simulink model "BuckyWagon_01"  (Simulink 7.5)
settings: Solver=FixedStepDiscrete  StartTime=0.0  StopTime=10.0  RelTol=1e-3
PreLoadFcn:
  | try, eval([bdroot '_setup']); catch, eval('model_setup', ''); end
InitFcn:
  | try, eval([bdroot '_setup']); catch, eval('model_setup', ''); end
undefined symbols (not defined in the file): ECU565, High, Low, miniviewSetup, motohawk_build_version, motohawk_get_faults, motohawk_setup_toolchains, motohawk_trunc_name, motohawk_vardec_config_group, motohawk_vardec_path, tc, True
libraries: MotoHawk_lib x381, simulink x26, miniview_lib x10, motohawk_control_primitives_lib x8, motohawk_engine_lib x6, motohawk_annotations_lib x2
(part 3 of 6)

== system BuckyWagon_01/Strategy/Actuators/A123 Battery Controller ==
  Contactor Command : Inport  OutDataType=sfix(16)  OutScaling=2^0
  Compare To Constant : simulink/Logic and Bit Operations/Compare To Constant  SystemSampleTime=-1  relop=>=  const=5  LogicOutDataTypeMode=uint8
  Emergency Power Off Comand : Constant  Value=0  OutDataTypeMode=uint8  OutDataType=fixdt(1, 16)  OutScaling=2^0  OutDataTypeStr=uint8
  Main Enable : Constant  OutDataTypeMode=uint8  OutDataType=fixdt(1, 16)  OutScaling=2^0  OutDataTypeStr=uint8
  Send CAN Messages3 : MotoHawk_lib/CAN Blocks/Send CAN Messages  bus=-2  nam='CAN_2'  msgl=BMS_A123_400  pace=5  labelwires=off
  Time Since Enabled (With Input)1 : motohawk_control_primitives_lib/Time Since Enabled (With Input)1  SystemSampleTime=-1  nam='A123_GroundFaultDetector_Enable_Timer'  samp_time=-1  init=0  upperlim=3600*24
  motohawk_override_abs5 : MotoHawk_lib/Calibration & Probing Blocks/motohawk_override_abs  SystemSampleTime=-1  parent_name='hsc_bcm_enable'  parent_val=0  show_more=on  name_source=Use Parameter  parent_read_level=1  parent_override_level=1  view_as=Number  enum_struct={'Disabled', 'Enabled'}  use_help_units=off  parent_help=''  parent_units=''  use_min_max=off  parent_min=-inf  parent_max=inf  use_precision=off  parent_precision=''  parent_gain=1  parent_offset=0  parent_exp=1  use_mototune_group=on  parent_group='Actuators | BCM'
  motohawk_override_abs6 : MotoHawk_lib/Calibration & Probing Blocks/motohawk_override_abs  SystemSampleTime=-1  parent_name='hsc_bcm_epo'  parent_val=0  show_more=on  name_source=Use Parameter  parent_read_level=1  parent_override_level=1  view_as=Number  enum_struct={'Disabled', 'Enabled'}  use_help_units=off  parent_help=''  parent_units=''  use_min_max=off  parent_min=-inf  parent_max=inf  use_precision=off  parent_precision=''  parent_gain=1  parent_offset=0  parent_exp=1  use_mototune_group=on  parent_group='Actuators | BCM'
  motohawk_override_abs7 : MotoHawk_lib/Calibration & Probing Blocks/motohawk_override_abs  SystemSampleTime=-1  parent_name='hsc_bcm_leakage_enable'  parent_val=0  show_more=on  name_source=Use Parameter  parent_read_level=1  parent_override_level=1  view_as=Number  enum_struct={'Disabled', 'Enabled'}  use_help_units=off  parent_help=''  parent_units=''  use_min_max=off  parent_min=-inf  parent_max=inf  use_precision=off  parent_precision=''  parent_gain=1  parent_offset=0  parent_exp=1  use_mototune_group=on  parent_group='Actuators | BCM'
  motohawk_override_abs8 : MotoHawk_lib/Calibration & Probing Blocks/motohawk_override_abs  SystemSampleTime=-1  parent_name='hsc_bcm_mainc_enable'  parent_val=0  show_more=on  name_source=Use Parameter  parent_read_level=1  parent_override_level=1  view_as=Number  enum_struct={'Disabled', 'Enabled'}  use_help_units=off  parent_help=''  parent_units=''  use_min_max=off  parent_min=-inf  parent_max=inf  use_precision=off  parent_precision=''  parent_gain=1  parent_offset=0  parent_exp=1  use_mototune_group=on  parent_group='Actuators | BCM'
  motohawk_probe6 : MotoHawk_lib/Calibration & Probing Blocks/motohawk_probe  nam='hsc_bcm_enable'  show_more=on  name_source=Use Parameter  read_level=1  view_as=Number  enum_struct={'Disabled', 'Enabled'}  vector_style=Wide Row  use_help_units=off  help=''  units=''  use_header_enum=off  row_header_enum={}  col_header_enum={}  use_precision=off  precision=''  gain=1  offset=0  exp=1  use_mototune_group=on  mototune_group='Actuators | BCM'
  motohawk_probe7 : MotoHawk_lib/Calibration & Probing Blocks/motohawk_probe  nam='hsc_bcm_epo'  show_more=on  name_source=Use Parameter  read_level=1  view_as=Number  enum_struct={'Disabled', 'Enabled'}  vector_style=Wide Row  use_help_units=off  help=''  units=''  use_header_enum=off  row_header_enum={}  col_header_enum={}  use_precision=off  precision=''  gain=1  offset=0  exp=1  use_mototune_group=on  mototune_group='Actuators | BCM'
  motohawk_probe8 : MotoHawk_lib/Calibration & Probing Blocks/motohawk_probe  nam='hsc_bcm_leakage_enable'  show_more=on  name_source=Use Parameter  read_level=1  view_as=Number  enum_struct={'Disabled', 'Enabled'}  vector_style=Wide Row  use_help_units=off  help=''  units=''  use_header_enum=off  row_header_enum={}  col_header_enum={}  use_precision=off  precision=''  gain=1  offset=0  exp=1  use_mototune_group=on  mototune_group='Actuators | BCM'
  motohawk_probe9 : MotoHawk_lib/Calibration & Probing Blocks/motohawk_probe  nam='hsc_bcm_mainc_enable'  show_more=on  name_source=Use Parameter  read_level=1  view_as=Number  enum_struct={'Disabled', 'Enabled'}  vector_style=Wide Row  use_help_units=off  help=''  units=''  use_header_enum=off  row_header_enum={}  col_header_enum={}  use_precision=off  precision=''  gain=1  offset=0  exp=1  use_mototune_group=on  mototune_group='Actuators | BCM'
  wires:
  motohawk_override_abs5/1 -> Send CAN Messages3/1
  motohawk_override_abs6/1 -> Send CAN Messages3/2
  motohawk_override_abs7/1 -> Send CAN Messages3/3
  motohawk_override_abs8/1 -> Send CAN Messages3/4
  Main Enable/1 -> motohawk_override_abs5/1, motohawk_probe6/1
  Emergency Power Off Comand/1 -> motohawk_override_abs6/1, motohawk_probe7/1
  Contactor Command/1 -> motohawk_override_abs8/1, motohawk_probe9/1, Time Since Enabled (With Input)1/1
  Compare To Constant/1 -> motohawk_override_abs7/1, motohawk_probe8/1
  Time Since Enabled (With Input)1/1 -> Compare To Constant/1

== system BuckyWagon_01/Strategy/Actuators/Brusa Charger ==
  In1 : Inport  OutDataType=sfix(16)  OutScaling=2^0
  Bus Selector : BusSelector  OutputSignals=CAN_Enable,ClearErrorLatch,ControlPilotVentReq,MaxMainsCurrent,OutputVoltageCommand,OutputCurrentCommand
  Send CAN Messages : MotoHawk_lib/CAN Blocks/Send CAN Messages  bus=-2  nam=['CAN_' num2str(1)]  msgl=can_BRUSA_618  pace=5  labelwires=on
  motohawk_override_abs{,1..2,4} (4 alike) : MotoHawk_lib/Calibration & Probing Blocks/motohawk_override_abs  SystemSampleTime=-1  parent_name='Override_Absolute'  parent_val=0  show_more=on  name_source=Use Output Wire Name  parent_read_level=1  parent_override_level=1  view_as=Number  enum_struct={'Disabled', 'Enabled'}  use_help_units=off  parent_help=''  parent_units=''  use_min_max=off  parent_min=-inf  parent_max=inf  use_precision=off  parent_precision=''  parent_gain=1  parent_offset=0  parent_exp=1  use_mototune_group=on  parent_group='Actuators | Brusa'
  motohawk_override_abs3 : MotoHawk_lib/Calibration & Probing Blocks/motohawk_override_abs  SystemSampleTime=-1  parent_name='Override_Absolute'  parent_val=0  show_more=on  name_source=Use Output Wire Name  parent_read_level=1  parent_override_level=1  view_as=Enumeration  enum_struct={'No Ventilation', 'Ventilation'}  use_help_units=off  parent_help=''  parent_units=''  use_min_max=off  parent_min=-inf  parent_max=inf  use_precision=off  parent_precision=''  parent_gain=1  parent_offset=0  parent_exp=1  use_mototune_group=on  parent_group='Actuators | Brusa'
  motohawk_override_abs5 : MotoHawk_lib/Calibration & Probing Blocks/motohawk_override_abs  SystemSampleTime=-1  parent_name='Override_Absolute'  parent_val=0  show_more=on  name_source=Use Output Wire Name  parent_read_level=1  parent_override_level=1  view_as=Enumeration  enum_struct={'Disabled', 'Enabled'}  use_help_units=off  parent_help=''  parent_units=''  use_min_max=off  parent_min=-inf  parent_max=inf  use_precision=off  parent_precision=''  parent_gain=1  parent_offset=0  parent_exp=1  use_mototune_group=on  parent_group='Actuators | Brusa'
  motohawk_probe{,1..2,4} (4 alike) : MotoHawk_lib/Calibration & Probing Blocks/motohawk_probe  nam='Probe'  show_more=on  name_source=Use Input Wire Name  read_level=1  view_as=Number  enum_struct={'Disabled', 'Enabled'}  vector_style=Wide Row  use_help_units=off  help=''  units=''  use_header_enum=off  row_header_enum={}  col_header_enum={}  use_precision=off  precision=''  gain=1  offset=0  exp=1  use_mototune_group=on  mototune_group='Actuators | Brusa'
  motohawk_probe3 : MotoHawk_lib/Calibration & Probing Blocks/motohawk_probe  nam='Probe'  show_more=on  name_source=Use Input Wire Name  read_level=1  view_as=Enumeration  enum_struct={'No Ventilation', 'Ventilation'}  vector_style=Wide Row  use_help_units=off  help=''  units=''  use_header_enum=off  row_header_enum={}  col_header_enum={}  use_precision=off  precision=''  gain=1  offset=0  exp=1  use_mototune_group=on  mototune_group='Actuators | Brusa'
  motohawk_probe5 : MotoHawk_lib/Calibration & Probing Blocks/motohawk_probe  nam='Probe'  show_more=on  name_source=Use Input Wire Name  read_level=1  view_as=Enumeration  enum_struct={'Disabled', 'Enabled'}  vector_style=Wide Row  use_help_units=off  help=''  units=''  use_header_enum=off  row_header_enum={}  col_header_enum={}  use_precision=off  precision=''  gain=1  offset=0  exp=1  use_mototune_group=on  mototune_group='Actuators | Brusa'
  wires:
  motohawk_override_abs5/1 -> Send CAN Messages/1, motohawk_probe5/1  "CAN_Enable"
  motohawk_override_abs4/1 -> Send CAN Messages/2, motohawk_probe4/1  "ClearErrorLtch"
  motohawk_override_abs3/1 -> Send CAN Messages/3, motohawk_probe3/1  "CntrlPltVentReq"
  motohawk_override_abs2/1 -> Send CAN Messages/4, motohawk_probe2/1  "MaxMainsCrnt"
  motohawk_override_abs1/1 -> Send CAN Messages/5, motohawk_probe1/1  "OutVoltCmd"
  motohawk_override_abs/1 -> Send CAN Messages/6, motohawk_probe/1  "OutCrntCmd"
  Bus Selector/1 -> motohawk_override_abs5/1  "<CAN_Enable>"
  Bus Selector/2 -> motohawk_override_abs4/1  "<ClearErrorLatch>"
  Bus Selector/3 -> motohawk_override_abs3/1  "<ControlPilotVentReq>"
  Bus Selector/4 -> motohawk_override_abs2/1  "<MaxMainsCurrent>"
  Bus Selector/5 -> motohawk_override_abs1/1  "<OutputVoltageCommand>"
  Bus Selector/6 -> motohawk_override_abs/1  "<OutputCurrentCommand>"
  In1/1 -> Bus Selector/1

== system BuckyWagon_01/Strategy/Actuators/Cruise Control Indicator ==
  Chart : Stateflow chart  TreatAsAtomicUnit=on
  motohawk_calibration1 : MotoHawk_lib/Calibration & Probing Blocks/motohawk_calibration  nam='cCInd_ShortTime'  val=20  storage=Calibration  show_more=on  name_source=Use Parameter  data_type=uint16  read_level=1  write_level=1  ovr_cals=on  view_as=Number  enum_struct={'Disabled', 'Enabled'}  vector_style=Wide Row  use_help_units=on  help='Short Off time in sequence.'  units='s'  use_header_enum=off  row_header_enum={}  col_header_enum={}  use_min_max=on  min_val=0  max_val=100  use_precision=on  precision='1.3'  gain=0.005  offset=0  exp=1  use_mototune_group=off  mototune_group=motohawk_vardec_path(gcb)
  motohawk_calibration2 : MotoHawk_lib/Calibration & Probing Blocks/motohawk_calibration  nam='cCInd_LongOff'  val=300  storage=Calibration  show_more=on  name_source=Use Parameter  data_type=uint16  read_level=1  write_level=1  ovr_cals=on  view_as=Number  enum_struct={'Disabled', 'Enabled'}  vector_style=Wide Row  use_help_units=on  help='Long Off time in flash sequence.'  units='s'  use_header_enum=off  row_header_enum={}  col_header_enum={}  use_min_max=on  min_val=0  max_val=100  use_precision=on  precision='1.3'  gain=0.005  offset=0  exp=1  use_mototune_group=off  mototune_group=motohawk_vardec_path(gcb)
  motohawk_calibration3 : MotoHawk_lib/Calibration & Probing Blocks/motohawk_calibration  nam='cCInd_OnTime'  val=10  storage=Calibration  show_more=on  name_source=Use Parameter  data_type=uint16  read_level=1  write_level=1  ovr_cals=on  view_as=Number  enum_struct={'Disabled', 'Enabled'}  vector_style=Wide Row  use_help_units=on  help='On time in flash sequence.'  units='s'  use_header_enum=off  row_header_enum={}  col_header_enum={}  use_min_max=on  min_val=0  max_val=100  use_precision=on  precision='1.3'  gain=0.005  offset=0  exp=1  use_mototune_group=off  mototune_group=motohawk_vardec_path(gcb)
  motohawk_data_read : MotoHawk_lib/Data Storage Blocks/motohawk_data_read  source=Lookup By Name  structure=Scalar  operation=Read scalar from location by index  sz_vec=4  sz_row=2  sz_col=3  typ=uint8  nam='cCOn'  checkNull=on  struct_inst_name=''  struct_nam='MyStruct'
  Out : Outport  OutDataType=sfix(16)  OutScaling=2^0
  wires:
  motohawk_data_read/1 -> Chart/1(cCOn)
  motohawk_calibration2/1 -> Chart/2(offLongTime)
  motohawk_calibration1/1 -> Chart/3(offShortTime)
  motohawk_calibration3/1 -> Chart/4(onTime)
  Chart/1(light) -> Out/1

== system BuckyWagon_01/Strategy/Actuators/EHPAS Power Steering Pump Controller ==
  Enable : Inport  DataType=boolean  OutDataType=sfix(16)  OutScaling=2^0  OutDataTypeStr=boolean
  Operating Mode - Activate : Constant  OutDataTypeMode=uint8  OutDataType=sfix(16)  OutScaling=2^0  OutDataTypeStr=uint8
  Operating Mode - Disabled : Constant  Value=0  OutDataTypeMode=uint8  OutDataType=sfix(16)  OutScaling=2^0  OutDataTypeStr=uint8
  Send CAN Messages : MotoHawk_lib/CAN Blocks/Send CAN Messages  bus=-2  nam='CAN_2'  msgl=J1939_6A_PowerSteering_Control  pace=5  labelwires=off
  Switch : Switch  Criteria=u2 ~= 0  OutDataType=fixdt(1, 16)  OutScaling=2^0
  motohawk_calibration2 : MotoHawk_lib/Calibration & Probing Blocks/motohawk_calibration  nam='EHPAS_Performance_Limit'  val=100  storage=Calibration  show_more=on  name_source=Use Parameter  data_type=double  read_level=1  write_level=1  ovr_cals=on  view_as=Number  enum_struct={'Disabled', 'Enabled'}  vector_style=Wide Row  use_help_units=off  help=''  units=''  use_header_enum=off  row_header_enum={}  col_header_enum={}  use_min_max=off  min_val=-inf  max_val=inf  use_precision=off  precision=''  gain=1  offset=0  exp=1  use_mototune_group=on  mototune_group='Actuators | EHPAS'
  motohawk_override_abs4 : MotoHawk_lib/Calibration & Probing Blocks/motohawk_override_abs  SystemSampleTime=-1  parent_name='EHPAS_Operating_Mode_Cmd'  parent_val=0  show_more=on  name_source=Use Parameter  parent_read_level=1  parent_override_level=1  view_as=Number  enum_struct={'Disabled', 'Enabled'}  use_help_units=off  parent_help=''  parent_units=''  use_min_max=off  parent_min=-inf  parent_max=inf  use_precision=off  parent_precision=''  parent_gain=1  parent_offset=0  parent_exp=1  use_mototune_group=on  parent_group='Actuators | EHPAS'
  motohawk_probe5 : MotoHawk_lib/Calibration & Probing Blocks/motohawk_probe  nam='EHPAS_Operating_Mode_Command'  show_more=on  name_source=Use Parameter  read_level=1  view_as=Number  enum_struct={'Disabled', 'Enabled'}  vector_style=Wide Row  use_help_units=off  help=''  units=''  use_header_enum=off  row_header_enum={}  col_header_enum={}  use_precision=off  precision=''  gain=1  offset=0  exp=1  use_mototune_group=on  mototune_group='Actuators | EHPAS'
  wires:
  motohawk_calibration2/1 -> Send CAN Messages/2
  motohawk_override_abs4/1 -> Send CAN Messages/1  "EHPAS_Operating_Mode_Cmd"
  Enable/1 -> Switch/2
  Operating Mode - Activate/1 -> Switch/1
  Operating Mode - Disabled/1 -> Switch/3
  Switch/1 -> motohawk_override_abs4/1, motohawk_probe5/1  "OperatingMode_cmd"

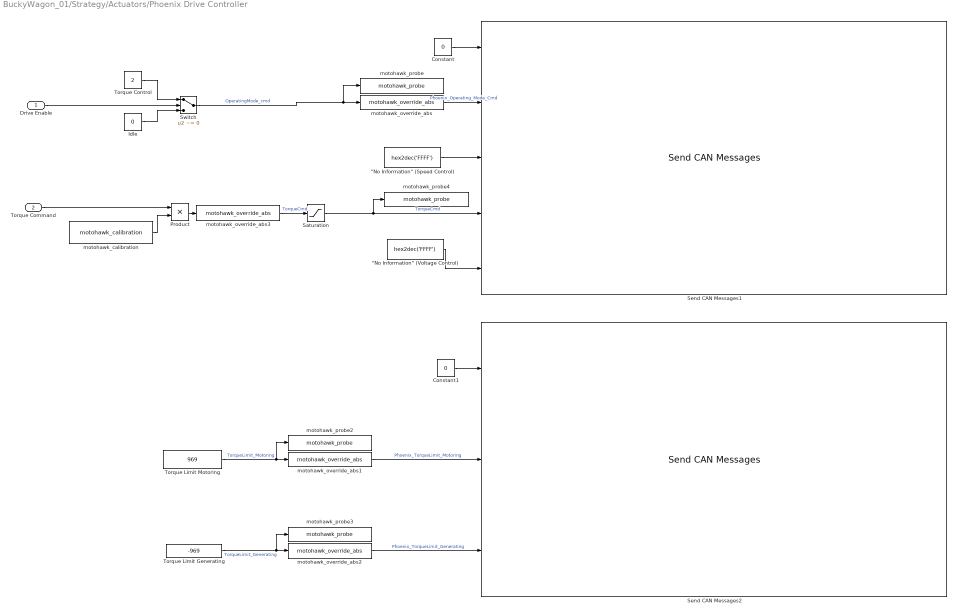
== system BuckyWagon_01/Strategy/Actuators/Phoenix Drive Controller ==
  Drive Enable : Inport  DataType=boolean  OutDataType=sfix(16)  OutScaling=2^0  OutDataTypeStr=boolean
  Torque Command : Inport  Port=2  OutDataType=sfix(16)  OutScaling=2^0
  "\"No Information\" (Speed Control)" : Constant  Value=hex2dec('FFFF')  OutDataTypeMode=uint16  OutDataType=sfix(16)  OutScaling=2^0  OutDataTypeStr=uint16
  "\"No Information\" (Voltage Control)" : Constant  Value=hex2dec('FFFF')  OutDataTypeMode=uint16  OutDataType=sfix(16)  OutScaling=2^0  OutDataTypeStr=uint16
  Constant : Constant  Value=0  OutDataType=sfix(16)  OutScaling=2^0
  Constant1 : Constant  Value=0  OutDataType=sfix(16)  OutScaling=2^0
  Idle : Constant  Value=0  OutDataType=sfix(16)  OutScaling=2^0
  Product : Product  OutDataType=sfix(16)  OutScaling=2^0  RndMeth=Zero
  Saturation : Saturate  UpperLimit=+3200  LowerLimit=-3200  OutDataType=fixdt(1, 16)  OutScaling=2^0
  Send CAN Messages1 : MotoHawk_lib/CAN Blocks/Send CAN Messages  bus=-2  nam='CAN_1'  msgl=J1939_F9_Control1  pace=5  labelwires=off
  Send CAN Messages2 : MotoHawk_lib/CAN Blocks/Send CAN Messages  bus=-2  nam='CAN_1'  msgl=J1939_F9_Control2  pace=5  labelwires=off
  Switch : Switch  Criteria=u2 ~= 0  OutDataType=fixdt(1, 16)  OutScaling=2^0
  Torque Control : Constant  Value=2  OutDataType=sfix(16)  OutScaling=2^0
  Torque Limit Generating : Constant  Value=-969  OutDataType=sfix(16)  OutScaling=2^0
  Torque Limit Motoring : Constant  Value=969  OutDataType=sfix(16)  OutScaling=2^0
  motohawk_calibration : MotoHawk_lib/Calibration & Probing Blocks/motohawk_calibration  nam='MaxTorque'  val=120  storage=Calibration  show_more=on  name_source=Use Parameter  data_type=Inherit from 'Default Value'  read_level=1  write_level=1  ovr_cals=on  view_as=Number  enum_struct={'Disabled', 'Enabled'}  vector_style=Wide Row  use_help_units=off  help=''  units=''  use_header_enum=off  row_header_enum={}  col_header_enum={}  use_min_max=off  min_val=-inf  max_val=inf  use_precision=off  precision=''  gain=1  offset=0  exp=1  use_mototune_group=on  mototune_group='Actuators | Phoenix'
  motohawk_override_abs : MotoHawk_lib/Calibration & Probing Blocks/motohawk_override_abs  SystemSampleTime=-1  parent_name='Override_Absolute'  parent_val=0  show_more=on  name_source=Use Output Wire Name  parent_read_level=1  parent_override_level=1  view_as=Number  enum_struct={'Disabled', 'Enabled'}  use_help_units=off  parent_help=''  parent_units=''  use_min_max=off  parent_min=-inf  parent_max=inf  use_precision=off  parent_precision=''  parent_gain=1  parent_offset=0  parent_exp=1  use_mototune_group=on  parent_group='Actuators | Phoenix'
  motohawk_override_abs1 : MotoHawk_lib/Calibration & Probing Blocks/motohawk_override_abs  SystemSampleTime=-1  parent_name='Override_Absolute'  parent_val=0  show_more=on  name_source=Use Output Wire Name  parent_read_level=1  parent_override_level=1  view_as=Number  enum_struct={'Disabled', 'Enabled'}  use_help_units=off  parent_help=''  parent_units=''  use_min_max=off  parent_min=-inf  parent_max=inf  use_precision=off  parent_precision=''  parent_gain=1  parent_offset=0  parent_exp=1  use_mototune_group=on  parent_group='Actuators | Phoenix'
  motohawk_override_abs2 : MotoHawk_lib/Calibration & Probing Blocks/motohawk_override_abs  SystemSampleTime=-1  parent_name='Override_Absolute'  parent_val=0  show_more=on  name_source=Use Output Wire Name  parent_read_level=1  parent_override_level=1  view_as=Number  enum_struct={'Disabled', 'Enabled'}  use_help_units=off  parent_help=''  parent_units=''  use_min_max=off  parent_min=-inf  parent_max=inf  use_precision=off  parent_precision=''  parent_gain=1  parent_offset=0  parent_exp=1  use_mototune_group=on  parent_group='Actuators | Phoenix'
  motohawk_override_abs3 : MotoHawk_lib/Calibration & Probing Blocks/motohawk_override_abs  SystemSampleTime=-1  parent_name='TorqueControl'  parent_val=0  show_more=on  name_source=Use Parameter  parent_read_level=1  parent_override_level=1  view_as=Number  enum_struct={'Disabled', 'Enabled'}  use_help_units=off  parent_help=''  parent_units=''  use_min_max=off  parent_min=-inf  parent_max=inf  use_precision=off  parent_precision=''  parent_gain=1  parent_offset=0  parent_exp=1  use_mototune_group=on  parent_group='Actuators | Phoenix'
  motohawk_probe : MotoHawk_lib/Calibration & Probing Blocks/motohawk_probe  nam='Phoenix_Operating_Mode_Command'  show_more=on  name_source=Use Parameter  read_level=1  view_as=Number  enum_struct={'Disabled', 'Enabled'}  vector_style=Wide Row  use_help_units=off  help=''  units=''  use_header_enum=off  row_header_enum={}  col_header_enum={}  use_precision=off  precision=''  gain=1  offset=0  exp=1  use_mototune_group=on  mototune_group='Actuators | Phoenix'
  motohawk_probe2 : MotoHawk_lib/Calibration & Probing Blocks/motohawk_probe  nam='Phoenix_TorqueLimit_Motoring'  show_more=on  name_source=Use Parameter  read_level=1  view_as=Number  enum_struct={'Disabled', 'Enabled'}  vector_style=Wide Row  use_help_units=off  help=''  units=''  use_header_enum=off  row_header_enum={}  col_header_enum={}  use_precision=off  precision=''  gain=1  offset=0  exp=1  use_mototune_group=on  mototune_group='Actuators | Phoenix'
  motohawk_probe3 : MotoHawk_lib/Calibration & Probing Blocks/motohawk_probe  nam='Phoenix_TorqueLimit_Generating'  show_more=on  name_source=Use Parameter  read_level=1  view_as=Number  enum_struct={'Disabled', 'Enabled'}  vector_style=Wide Row  use_help_units=off  help=''  units=''  use_header_enum=off  row_header_enum={}  col_header_enum={}  use_precision=off  precision=''  gain=1  offset=0  exp=1  use_mototune_group=on  mototune_group='Actuators | Phoenix'
  motohawk_probe4 : MotoHawk_lib/Calibration & Probing Blocks/motohawk_probe  nam='Phoenix_TorqueCmd_final'  show_more=on  name_source=Use Parameter  read_level=1  view_as=Number  enum_struct={'Disabled', 'Enabled'}  vector_style=Wide Row  use_help_units=off  help=''  units=''  use_header_enum=off  row_header_enum={}  col_header_enum={}  use_precision=off  precision=''  gain=1  offset=0  exp=1  use_mototune_group=on  mototune_group='Actuators | Phoenix'
  wires:
  Torque Command/1 -> Product/1
  motohawk_override_abs/1 -> Send CAN Messages1/2  "Phoenix_Operating_Mode_Cmd"
  Switch/1 -> motohawk_override_abs/1, motohawk_probe/1  "OperatingMode_cmd"
  motohawk_calibration/1 -> Product/2
  Product/1 -> motohawk_override_abs3/1
  "\"No Information\" (Speed Control)"/1 -> Send CAN Messages1/3
  "\"No Information\" (Voltage Control)"/1 -> Send CAN Messages1/5
  motohawk_override_abs3/1 -> Saturation/1  "TorqueCmd"
  Saturation/1 -> Send CAN Messages1/4, motohawk_probe4/1  "TorqueCmd"
  motohawk_override_abs1/1 -> Send CAN Messages2/2  "Phoenix_TorqueLimit_Motoring"
  Torque Limit Motoring/1 -> motohawk_probe2/1, motohawk_override_abs1/1  "TorqueLimit_Motoring"
  motohawk_override_abs2/1 -> Send CAN Messages2/3  "Phoenix_TorqueLimit_Generating"
  Torque Limit Generating/1 -> motohawk_override_abs2/1, motohawk_probe3/1  "TorqueLimit_Generating"
  Drive Enable/1 -> Switch/2
  Idle/1 -> Switch/3
  Torque Control/1 -> Switch/1
  Constant/1 -> Send CAN Messages1/1
  Constant1/1 -> Send CAN Messages2/1

== system BuckyWagon_01/Strategy/Actuators/ReverseInd ==
  In : Inport  OutDataType=sfix(16)  OutScaling=2^0
  Enabled Subsystem : Subsystem  TreatAsAtomicUnit=on
  Logical Operator : Logic  IconShape=distinctive  AllPortsSameDT=off  OutDataTypeMode=boolean  OutDataTypeStr=boolean
  Logical Operator1 : Logic  AllPortsSameDT=off  OutDataTypeMode=boolean  OutDataTypeStr=boolean
  Logical Operator2 : Logic  Operator=OR  AllPortsSameDT=off  OutDataTypeMode=boolean  OutDataTypeStr=boolean
  Logical Operator3 : Logic  IconShape=distinctive  AllPortsSameDT=off  OutDataTypeMode=boolean  OutDataTypeStr=boolean
  Logical Operator4 : Logic  Operator=NOT  IconShape=distinctive  AllPortsSameDT=off  OutDataTypeMode=boolean  OutDataTypeStr=boolean
  motohawk_calibration1 : MotoHawk_lib/Calibration & Probing Blocks/motohawk_calibration  nam='RevIndType'  val=1  storage=Calibration  show_more=on  name_source=Use Parameter  data_type=uint8  read_level=1  write_level=1  ovr_cals=on  view_as=Enumeration  enum_struct={'Flash', 'Solid'}  vector_style=Wide Row  use_help_units=on  help='Mode for Reverse Indicator'  units=''  use_header_enum=off  row_header_enum={}  col_header_enum={}  use_min_max=on  min_val=0  max_val=100  use_precision=on  precision=''  gain=1  offset=0  exp=1  use_mototune_group=off  mototune_group=motohawk_vardec_path(gcb)
  motohawk_calibration2 : MotoHawk_lib/Calibration & Probing Blocks/motohawk_calibration  nam='ReverseIndFlash_Period'  val=150  storage=Calibration  show_more=on  name_source=Use Parameter  data_type=int16  read_level=1  write_level=1  ovr_cals=on  view_as=Number  enum_struct={'Disabled', 'Enabled'}  vector_style=Wide Row  use_help_units=on  help='Period for the flashing reverse indicator.'  units='s'  use_header_enum=off  row_header_enum={}  col_header_enum={}  use_min_max=on  min_val=0  max_val=100  use_precision=on  precision='1.3'  gain=0.005  offset=0  exp=1  use_mototune_group=off  mototune_group=motohawk_vardec_path(gcb)
  Out : Outport  OutDataType=sfix(16)  OutScaling=2^0
  wires:
  Logical Operator1/1 -> Logical Operator2/2
  Enabled Subsystem/1(Out) -> Logical Operator1/2
  Logical Operator2/1 -> Out/1
  motohawk_calibration2/1 -> Enabled Subsystem/1(Period (Cnt))
  Logical Operator3/1 -> Enabled Subsystem/Enable, Logical Operator1/1
  Logical Operator/1 -> Logical Operator2/1
  motohawk_calibration1/1 -> Logical Operator/1, Logical Operator4/1
  Logical Operator4/1 -> Logical Operator3/2
  In/1 -> Logical Operator/2, Logical Operator3/1

== system BuckyWagon_01/Strategy/Control Strategy/Assist ==
  Inputs : Inport  OutDataType=sfix(16)  OutScaling=2^0
  Bus Selector1 : BusSelector  OutputSignals=Accel
  Constant3 : Constant  OutDataType=sfix(16)  OutScaling=2^0
  CruiseControl : Subsystem  TreatAsAtomicUnit=on
  Saturation Dynamic : simulink/Discontinuities/Saturation Dynamic  SystemSampleTime=-1  OutMin=[]  OutMax=[]  OutDataTypeStr=Inherit: Same as second input  OutDataType=sfix(16)  OutScaling=2^-10  DoSatur=off
  Saturation1 : Saturate  UpperLimit=1  LowerLimit=0
  StallTorqueFault : Subsystem
  motohawk_table_1d : MotoHawk_lib/Lookup Tables/motohawk_table_1d  SystemSampleTime=-1  nam='AccelTorqueMap'  bp_nam=''  breakpoint_data=[0 0.1 0.2 0.3 0.4 0.5 0.6 0.7 0.8 0.9 1]  table_data=[0 0.1 0.2 0.3 0.4 0.5 0.6 0.7 0.8 0.9 1]  show_more=on  bp_data_type=Inherit from 'Breakpoint Data'  bp_storage=Constant  table_data_type=Inherit from 'Table Data'  storage=NonAdaptive  read_level=1  write_level=1  ovr_cals=on  use_help=off  help=''  bp_units=''  table_units=''  use_min_max=on  bp_min_val=0  bp_max_val=1  min_val=-inf  max_val=inf  use_precision=off  use_breakpoint=off  b_precision=''  b_gain=1  b_offset=0  b_exp=1  use_table=off  t_precision=''  t_gain=1  t_offset=0  t_exp=1  use_links=off  input_name=''  output_name=''  use_mototune_group=off  mototune_group=motohawk_vardec_path(gcb)
  Outputs : Outport  OutDataType=sfix(16)  OutScaling=2^0
  wires:
  Saturation1/1 -> Outputs/1, StallTorqueFault/2(Torque)  "motor_Torque"
  Inputs/1 -> Bus Selector1/1, CruiseControl/1(Inputs), StallTorqueFault/1(Inputs)
  Bus Selector1/1 -> motohawk_table_1d/1  "<Accel>"
  motohawk_table_1d/1 -> Saturation Dynamic/2
  Saturation Dynamic/1 -> Saturation1/1
  CruiseControl/1(Outputs) -> Saturation Dynamic/3
  Constant3/1 -> Saturation Dynamic/1

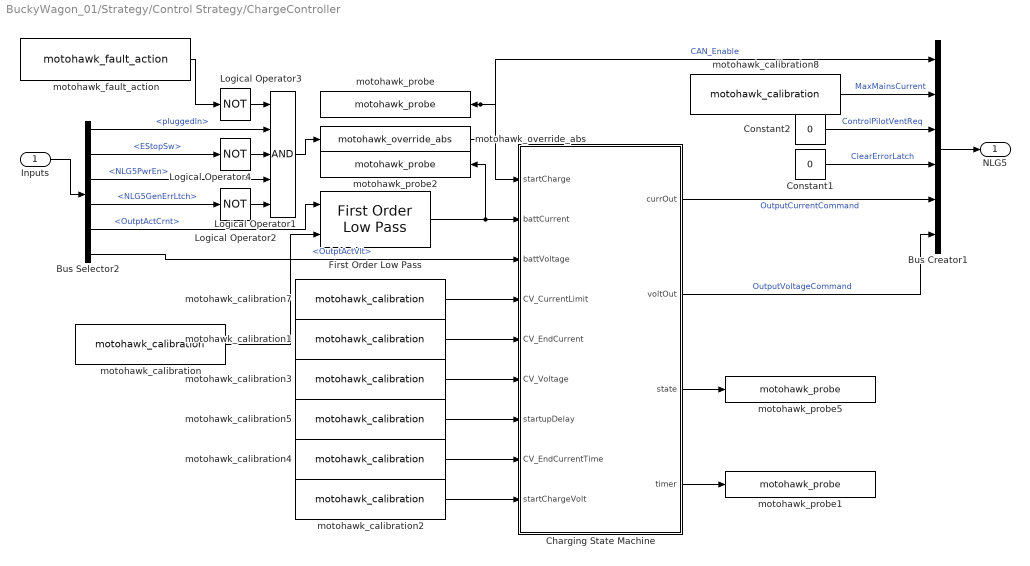
== system BuckyWagon_01/Strategy/Control Strategy/ChargeController ==
  Inputs : Inport  OutDataType=sfix(16)  OutScaling=2^0
  Bus Creator1 : BusCreator  Inputs=6
  Bus Selector2 : BusSelector  OutputSignals=NLG5.pluggedIn,EStopSw,NLG5.Status.NLG5PwrEn,NLG5.Status.NLG5GenErrLtch,NLG5.ActualValues1.OutptActCrnt,NLG5.ActualValues1.OutptActVlt
  Charging State Machine : Stateflow chart  TreatAsAtomicUnit=on
  Constant1 : Constant  Value=0  OutDataTypeMode=uint8  OutDataType=sfix(16)  OutScaling=2^0  OutDataTypeStr=uint8
  Constant2 : Constant  Value=0  OutDataTypeMode=uint8  OutDataType=sfix(16)  OutScaling=2^0  OutDataTypeStr=uint8
  First Order Low Pass : motohawk_control_primitives_lib/First Order Low Pass  SystemSampleTime=-1
  Logical Operator1 : Logic  Inputs=5  AllPortsSameDT=off  OutDataTypeMode=boolean  OutDataTypeStr=boolean
  Logical Operator2 : Logic  Operator=NOT  AllPortsSameDT=off  OutDataTypeMode=boolean  OutDataTypeStr=boolean
  Logical Operator3 : Logic  Operator=NOT  AllPortsSameDT=off  OutDataTypeMode=boolean  OutDataTypeStr=boolean
  Logical Operator4 : Logic  Operator=NOT  AllPortsSameDT=off  OutDataTypeMode=boolean  OutDataTypeStr=boolean
  motohawk_calibration : MotoHawk_lib/Calibration & Probing Blocks/motohawk_calibration  nam='IFilterAlpha'  val=0.01  storage=Calibration  show_more=on  name_source=Use Parameter  data_type=Inherit from 'Default Value'  read_level=1  write_level=1  ovr_cals=on  view_as=Number  enum_struct={'Disabled', 'Enabled'}  vector_style=Wide Row  use_help_units=off  help=''  units=''  use_header_enum=off  row_header_enum={}  col_header_enum={}  use_min_max=on  min_val=0  max_val=1  use_precision=on  precision='1.4'  gain=1  offset=0  exp=1  use_mototune_group=off  mototune_group=motohawk_vardec_path(gcb)
  motohawk_calibration1 : MotoHawk_lib/Calibration & Probing Blocks/motohawk_calibration  nam='CV_EndCurrent'  val=2  storage=Calibration  show_more=on  name_source=Use Parameter  data_type=double  read_level=1  write_level=1  ovr_cals=on  view_as=Number  enum_struct={'Disabled', 'Enabled'}  vector_style=Wide Row  use_help_units=on  help='Below this current the charge is complete'  units='A'  use_header_enum=off  row_header_enum={}  col_header_enum={}  use_min_max=off  min_val=0  max_val=500  use_precision=on  precision='3.1'  gain=1  offset=0  exp=1  use_mototune_group=off  mototune_group=motohawk_vardec_path(gcb)
  motohawk_calibration2 : MotoHawk_lib/Calibration & Probing Blocks/motohawk_calibration  nam='restartChargeVolt'  val=350  storage=Calibration  show_more=on  name_source=Use Parameter  data_type=double  read_level=1  write_level=1  ovr_cals=on  view_as=Number  enum_struct={'Disabled', 'Enabled'}  vector_style=Wide Row  use_help_units=on  help='Below this voltage a completed charge will restart.'  units='V'  use_header_enum=off  row_header_enum={}  col_header_enum={}  use_min_max=off  min_val=0  max_val=500  use_precision=on  precision='3.1'  gain=1  offset=0  exp=1  use_mototune_group=off  mototune_group=motohawk_vardec_path(gcb)
  motohawk_calibration3 : MotoHawk_lib/Calibration & Probing Blocks/motohawk_calibration  nam='CV_Voltage'  val=372  storage=Calibration  show_more=on  name_source=Use Parameter  data_type=double  read_level=1  write_level=1  ovr_cals=on  view_as=Number  enum_struct={'Disabled', 'Enabled'}  vector_style=Wide Row  use_help_units=on  help='Commanded voltage during CV charge.'  units='V'  use_header_enum=off  row_header_enum={}  col_header_enum={}  use_min_max=off  min_val=0  max_val=500  use_precision=on  precision='3.1'  gain=1  offset=0  exp=1  use_mototune_group=off  mototune_group=motohawk_vardec_path(gcb)
  motohawk_calibration4 : MotoHawk_lib/Calibration & Probing Blocks/motohawk_calibration  nam='CV_EndCurrentTime'  val=3000  storage=Calibration  show_more=on  name_source=Use Parameter  data_type=uint16  read_level=1  write_level=1  ovr_cals=on  view_as=Number  enum_struct={'Disabled', 'Enabled'}  vector_style=Wide Row  use_help_units=on  help='Current must be below end limit this long to end charge.'  units='s'  use_header_enum=off  row_header_enum={}  col_header_enum={}  use_min_max=off  min_val=0  max_val=500  use_precision=on  precision='3.1'  gain=0.005  offset=0  exp=1  use_mototune_group=off  mototune_group=motohawk_vardec_path(gcb)
  motohawk_calibration5 : MotoHawk_lib/Calibration & Probing Blocks/motohawk_calibration  nam='ChargeStartupDelay'  val=400  storage=Calibration  show_more=on  name_source=Use Parameter  data_type=uint16  read_level=1  write_level=1  ovr_cals=on  view_as=Number  enum_struct={'Disabled', 'Enabled'}  vector_style=Wide Row  use_help_units=on  help='Charge will start after conditions met for this long.'  units='s'  use_header_enum=off  row_header_enum={}  col_header_enum={}  use_min_max=off  min_val=0  max_val=500  use_precision=on  precision='1.2'  gain=0.005  offset=0  exp=1  use_mototune_group=off  mototune_group=motohawk_vardec_path(gcb)
  motohawk_calibration7 : MotoHawk_lib/Calibration & Probing Blocks/motohawk_calibration  nam='CV_CurrentLimit'  val=10  storage=Calibration  show_more=on  name_source=Use Parameter  data_type=double  read_level=1  write_level=1  ovr_cals=on  view_as=Number  enum_struct={'Disabled', 'Enabled'}  vector_style=Wide Row  use_help_units=on  help='Current limit during CV charge.'  units='A'  use_header_enum=off  row_header_enum={}  col_header_enum={}  use_min_max=off  min_val=0  max_val=500  use_precision=on  precision='3.2'  gain=1  offset=0  exp=1  use_mototune_group=off  mototune_group=motohawk_vardec_path(gcb)
  motohawk_calibration8 : MotoHawk_lib/Calibration & Probing Blocks/motohawk_calibration  nam='MaxMainsCurrent'  val=16  storage=Calibration  show_more=on  name_source=Use Parameter  data_type=Inherit via back propagation  read_level=1  write_level=1  ovr_cals=on  view_as=Number  enum_struct={'Disabled', 'Enabled'}  vector_style=Wide Row  use_help_units=on  help='Maximum Mains Current the charger can draw'  units='A'  use_header_enum=off  row_header_enum={}  col_header_enum={}  use_min_max=on  min_val=0  max_val=50  use_precision=off  precision=''  gain=1  offset=0  exp=1  use_mototune_group=off  mototune_group=motohawk_vardec_path(gcb)
  motohawk_fault_action : MotoHawk_lib/Fault Management Blocks/motohawk_fault_action  nam='Charge_Fault'  output_status=on  eval_nam=Charge_Fault
  motohawk_override_abs : MotoHawk_lib/Calibration & Probing Blocks/motohawk_override_abs  SystemSampleTime=-1  parent_name='startCharge'  parent_val=0  show_more=off  name_source=Use Parameter  parent_read_level=1  parent_override_level=1  view_as=Number  enum_struct={'Disabled', 'Enabled'}  use_help_units=off  parent_help=''  parent_units=''  use_min_max=off  parent_min=-inf  parent_max=inf  use_precision=off  parent_precision=''  parent_gain=1  parent_offset=0  parent_exp=1  use_mototune_group=off  parent_group=motohawk_vardec_path(gcb)
  motohawk_probe : MotoHawk_lib/Calibration & Probing Blocks/motohawk_probe  nam='startCharge'  show_more=off  name_source=Use Parameter  read_level=1  view_as=Number  enum_struct={'Disabled', 'Enabled'}  vector_style=Wide Row  use_help_units=off  help=''  units=''  use_header_enum=off  row_header_enum={}  col_header_enum={}  use_precision=off  precision=''  gain=1  offset=0  exp=1  use_mototune_group=off  mototune_group=motohawk_vardec_path(gcb)
  motohawk_probe1 : MotoHawk_lib/Calibration & Probing Blocks/motohawk_probe  nam='ChargingTimer'  show_more=on  name_source=Use Parameter  read_level=1  view_as=Number  enum_struct={'WaitStart', 'CnstVolt', 'EndCnstVolt','Complete'}  vector_style=Wide Row  use_help_units=off  help=''  units=''  use_header_enum=off  row_header_enum={}  col_header_enum={}  use_precision=on  precision='1.2'  gain=0.005  offset=0  exp=1  use_mototune_group=off  mototune_group=motohawk_vardec_path(gcb)
  motohawk_probe2 : MotoHawk_lib/Calibration & Probing Blocks/motohawk_probe  nam='filteredCurrent'  show_more=off  name_source=Use Parameter  read_level=1  view_as=Number  enum_struct={'Disabled', 'Enabled'}  vector_style=Wide Row  use_help_units=off  help=''  units=''  use_header_enum=off  row_header_enum={}  col_header_enum={}  use_precision=off  precision=''  gain=1  offset=0  exp=1  use_mototune_group=off  mototune_group=motohawk_vardec_path(gcb)
  motohawk_probe5 : MotoHawk_lib/Calibration & Probing Blocks/motohawk_probe  nam='ChargingState'  show_more=on  name_source=Use Parameter  read_level=1  view_as=Enumeration  enum_struct={'Wait', 'CnstVolt', 'EndCnstVolt','Complete', 'delay'}  vector_style=Wide Row  use_help_units=off  help=''  units=''  use_header_enum=off  row_header_enum={}  col_header_enum={}  use_precision=off  precision=''  gain=1  offset=0  exp=1  use_mototune_group=off  mototune_group=motohawk_vardec_path(gcb)
  NLG5 : Outport  OutDataType=sfix(16)  OutScaling=2^0
  wires:
  Constant2/1 -> Bus Creator1/3  "ControlPilotVentReq"
  motohawk_calibration8/1 -> Bus Creator1/2  "MaxMainsCurrent"
  Constant1/1 -> Bus Creator1/4  "ClearErrorLatch"
  Charging State Machine/1(currOut) -> Bus Creator1/5  "OutputCurrentCommand"
  Charging State Machine/2(voltOut) -> Bus Creator1/6  "OutputVoltageCommand"
  Logical Operator1/1 -> motohawk_override_abs/1
  Logical Operator2/1 -> Logical Operator1/5
  Charging State Machine/3(state) -> motohawk_probe5/1
  Inputs/1 -> Bus Selector2/1
  Bus Selector2/4 -> Logical Operator2/1  "<NLG5GenErrLtch>"
  Bus Selector2/1 -> Logical Operator1/2  "<pluggedIn>"
  Bus Creator1/1 -> NLG5/1
  Charging State Machine/4(timer) -> motohawk_probe1/1
  motohawk_calibration7/1 -> Charging State Machine/4(CV_CurrentLimit)
  motohawk_calibration1/1 -> Charging State Machine/5(CV_EndCurrent)
  motohawk_calibration3/1 -> Charging State Machine/6(CV_Voltage)
  motohawk_calibration5/1 -> Charging State Machine/7(startupDelay)
  motohawk_calibration4/1 -> Charging State Machine/8(CV_EndCurrentTime)
  Bus Selector2/6 -> Charging State Machine/3(battVoltage)  "<OutptActVlt>"
  motohawk_calibration2/1 -> Charging State Machine/9(startChargeVolt)
  motohawk_override_abs/1 -> Charging State Machine/1(startCharge), Bus Creator1/1, motohawk_probe/1  "CAN_Enable"
  motohawk_fault_action/1 -> Logical Operator3/1
  Logical Operator3/1 -> Logical Operator1/1
  First Order Low Pass/1 -> Charging State Machine/2(battCurrent), motohawk_probe2/1
  Bus Selector2/5 -> First Order Low Pass/1  "<OutptActCrnt>"
  motohawk_calibration/1 -> First Order Low Pass/2
  Bus Selector2/2 -> Logical Operator4/1  "<EStopSw>"
  Logical Operator4/1 -> Logical Operator1/3
  Bus Selector2/3 -> Logical Operator1/4  "<NLG5PwrEn>"

== system BuckyWagon_01/Strategy/Control Strategy/HV Controller ==
  Battery Ready : Inport  OutDataType=sfix(16)  OutScaling=2^0
  Contactor Status : Inport  Port=2  OutDataType=sfix(16)  OutScaling=2^0
  Battery has passed power-on-self-test and is ready : simulink/Logic and Bit Operations/Compare To Constant  SystemSampleTime=-1  relop===  const=1  LogicOutDataTypeMode=boolean
  Constant : Constant  Value=0  OutDataType=fixdt(1, 16)  OutScaling=2^0
  Contacter Controller : Subsystem
  Contactors are closed and ready : simulink/Logic and Bit Operations/Compare To Constant  SystemSampleTime=-1  relop===  const=1  LogicOutDataTypeMode=boolean
  Logical Operator2 : Logic  Operator=OR  Inputs=3  AllPortsSameDT=off  OutDataTypeMode=boolean  OutDataTypeStr=boolean
  motohawk_data_read : MotoHawk_lib/Data Storage Blocks/motohawk_data_read  source=Lookup By Name  structure=Scalar  operation=Read scalar from location by index  sz_vec=4  sz_row=2  sz_col=3  typ=boolean  nam='Shutdown_Req'  checkNull=on  struct_inst_name='Struct1'  struct_nam='MyStruct'
  motohawk_fault_action : MotoHawk_lib/Fault Management Blocks/motohawk_fault_action  nam='EmergencyShutdown'  output_status=on  eval_nam=EmergencyShutdown
  motohawk_override_abs2 : MotoHawk_lib/Calibration & Probing Blocks/motohawk_override_abs  SystemSampleTime=-1  parent_name='Override_Absolute'  parent_val=0  show_more=on  name_source=Use Input Wire Name  parent_read_level=1  parent_override_level=1  view_as=Number  enum_struct={'Disabled', 'Enabled'}  use_help_units=off  parent_help=''  parent_units=''  use_min_max=on  parent_min=0  parent_max=1  use_precision=off  parent_precision=''  parent_gain=1  parent_offset=0  parent_exp=1  use_mototune_group=on  parent_group='BuckyWagon_01 | Strategy | Control Strategy | HV Controller'
  Contactor Command : Outport  OutDataType=sfix(16)  OutScaling=2^0
  Phoenix/Drive Enable : Outport  Port=2  OutDataType=sfix(16)  OutScaling=2^0
  Power Steering Pump Enable : Outport  Port=3  OutDataType=sfix(16)  OutScaling=2^0
  wires:
  Battery Ready/1 -> Battery has passed power-on-self-test and is ready/1
  Contacter Controller/1(Contactor_Enable) -> Contactor Command/1
  Contacter Controller/2(Load_Enable) -> Phoenix/Drive Enable/1, Power Steering Pump Enable/1
  Contactor Status/1 -> Contactors are closed and ready/1
  Battery has passed power-on-self-test and is ready/1 -> Contacter Controller/1(Battery OK)
  motohawk_fault_action/1 -> Logical Operator2/2
  motohawk_data_read/1 -> Logical Operator2/1
  Logical Operator2/1 -> Contacter Controller/2(Shutdown Command)
  Contactors are closed and ready/1 -> Contacter Controller/3(Contactor Status)
  motohawk_override_abs2/1 -> Logical Operator2/3
  Constant/1 -> motohawk_override_abs2/1  "Shutdown_Test"

== system BuckyWagon_01/Strategy/Control Strategy/Regen ==
  Inputs : Inport  OutDataType=sfix(16)  OutScaling=2^0
  Bus Selector1 : BusSelector  OutputSignals=BrakeSw
  Bus Selector2 : BusSelector  OutputSignals=VehicleSpeed,SOC
  Constant : Constant  Value=0  OutDataType=sfix(16)  OutScaling=2^0
  Gain1 : Gain  Gain=-1  ParameterDataType=sfix(16)  ParameterScaling=2^0  OutDataType=sfix(16)  OutScaling=2^0
  Multiport Switch : MultiPortSwitch  DataPortOrder=Zero-based contiguous  Inputs=2  zeroidx=on
  SOC_RampOut : Subsystem
  Saturation1 : motohawk_control_primitives_lib/Saturation  SystemSampleTime=-1
  Sum : Sum  Inputs=|++  OutDataType=sfix(16)  OutScaling=2^0
  Unit Delay : UnitDelay  SampleTime=-1
  motohawk_calibration1 : MotoHawk_lib/Calibration & Probing Blocks/motohawk_calibration  nam='RampOut_Rate'  val=0  storage=Calibration  show_more=on  name_source=Use Parameter  data_type=Inherit from 'Default Value'  read_level=1  write_level=1  ovr_cals=on  view_as=Number  enum_struct={'Disabled', 'Enabled'}  vector_style=Wide Row  use_help_units=on  help='Rate at which regen ramps out'  units='%/5ms'  use_header_enum=off  row_header_enum={}  col_header_enum={}  use_min_max=off  min_val=0  max_val=2  use_precision=on  precision='1.3'  gain=1  offset=0  exp=1  use_mototune_group=off  mototune_group=motohawk_vardec_path(gcb)
  motohawk_calibration2 : MotoHawk_lib/Calibration & Probing Blocks/motohawk_calibration  nam='RampIn_Rate'  val=0  storage=Calibration  show_more=on  name_source=Use Parameter  data_type=Inherit from 'Default Value'  read_level=1  write_level=1  ovr_cals=on  view_as=Number  enum_struct={'Disabled', 'Enabled'}  vector_style=Wide Row  use_help_units=off  help='Rate at which regen ramps in'  units='%/5ms'  use_header_enum=off  row_header_enum={}  col_header_enum={}  use_min_max=off  min_val=0  max_val=2  use_precision=on  precision='1.3'  gain=1  offset=0  exp=1  use_mototune_group=off  mototune_group=motohawk_vardec_path(gcb)
  motohawk_calibration3 : MotoHawk_lib/Calibration & Probing Blocks/motohawk_calibration  nam='RegenFull_Level'  val=0  storage=Calibration  show_more=on  name_source=Use Parameter  data_type=Inherit from 'Default Value'  read_level=1  write_level=1  ovr_cals=on  view_as=Number  enum_struct={'Disabled', 'Enabled'}  vector_style=Wide Row  use_help_units=on  help='Maximum Regen Level'  units='%'  use_header_enum=off  row_header_enum={}  col_header_enum={}  use_min_max=on  min_val=-1  max_val=0  use_precision=on  precision='1.3'  gain=1  offset=0  exp=1  use_mototune_group=off  mototune_group=motohawk_vardec_path(gcb)
  motohawk_data_def2 : MotoHawk_lib/Data Storage Blocks/motohawk_data_def  nam='Regen_Start'  container_nam=''  data=0  typ=double  struct_nam='MyStruct'  storage=NonVolatile  outputRef=off  use_vardec=on  window=Calibration  read_level=1  write_level=1  ovr_cals=on  view_as=Number  enum_struct={'Disabled', 'Enabled'}  vector_style=Wide Row  use_help_units=off  help='Regen Starts above this position'  units='%'  use_header_enum=off  row_header_enum=''  col_header_enum=''  use_min_max=off  min_val=0  max_val=1  use_precision=off  precision='1.2'  gain=1  offset=0  exp=1  use_mototune_group=off  mototune_group=motohawk_vardec_path(gcb)  eval_name=Regen_Start  data_stores=motohawk_sfun_data_def_data_stores  struct_instances=motohawk_sfun_data_def_struct_instances  vardecs=motohawk_sfun_data_def_vardecs
  motohawk_probe : MotoHawk_lib/Calibration & Probing Blocks/motohawk_probe  nam='Regen_Level_Ramp'  show_more=on  name_source=Use Parameter  read_level=1  view_as=Number  enum_struct={'Disabled', 'Enabled'}  vector_style=Wide Row  use_help_units=off  help=''  units=''  use_header_enum=off  row_header_enum={}  col_header_enum={}  use_precision=on  precision='1.2'  gain=1  offset=0  exp=1  use_mototune_group=off  mototune_group=motohawk_vardec_path(gcb)
  motohawk_probe1 : MotoHawk_lib/Calibration & Probing Blocks/motohawk_probe  nam='Regen_Level_Speed'  show_more=on  name_source=Use Parameter  read_level=1  view_as=Number  enum_struct={'Disabled', 'Enabled'}  vector_style=Wide Row  use_help_units=off  help=''  units=''  use_header_enum=off  row_header_enum={}  col_header_enum={}  use_precision=on  precision='1.2'  gain=1  offset=0  exp=1  use_mototune_group=off  mototune_group=motohawk_vardec_path(gcb)
  motohawk_probe2 : MotoHawk_lib/Calibration & Probing Blocks/motohawk_probe  nam='Regen_Level'  show_more=on  name_source=Use Parameter  read_level=1  view_as=Number  enum_struct={'Disabled', 'Enabled'}  vector_style=Wide Row  use_help_units=off  help=''  units=''  use_header_enum=off  row_header_enum={}  col_header_enum={}  use_precision=on  precision='1.2'  gain=1  offset=0  exp=1  use_mototune_group=off  mototune_group=motohawk_vardec_path(gcb)
  speed_RampOut : Subsystem
  Outputs : Outport  OutDataType=sfix(16)  OutScaling=2^0
  wires:
  Sum/1 -> Saturation1/1
  Unit Delay/1 -> Sum/2
  Multiport Switch/1 -> Sum/1
  Gain1/1 -> Multiport Switch/3
  motohawk_calibration1/1 -> Multiport Switch/2
  Bus Selector1/1 -> Multiport Switch/1  "<BrakeSw>"
  motohawk_calibration2/1 -> Gain1/1
  SOC_RampOut/1(Torque_Out) -> motohawk_probe2/1, Outputs/1  "motor_Torque"
  Bus Selector2/1 -> speed_RampOut/2(speed)  "<VehicleSpeed>"
  Bus Selector2/2 -> SOC_RampOut/2(SOC)  "<SOC>"
  speed_RampOut/1(Torque_Out) -> motohawk_probe1/1, SOC_RampOut/1(Torque_In)
  Saturation1/1 -> Unit Delay/1, motohawk_probe/1, speed_RampOut/1(Torque_In)  "motor_Torque"
  Inputs/1 -> Bus Selector1/1, Bus Selector2/1
  motohawk_calibration3/1 -> Saturation1/2
  Constant/1 -> Saturation1/3
